simulink model "heli0519"  (R2022a)
settings: Solver=VariableStepAuto  StartTime=0.0  StopTime=5.0  RelTol=1e-3
settings Model: Creator=jixiang  LastModifiedBy=kcx06
settings SolverCC: AlgebraicLoopSolver=TrustRegion
settings DebuggingCC: UnconnectedInputMsg=warning  UnconnectedOutputMsg=warning  UnconnectedLineMsg=warning  SFMachineParentedDataDiag=warning
settings RTWCC: DLArmComputeVersion=19.05

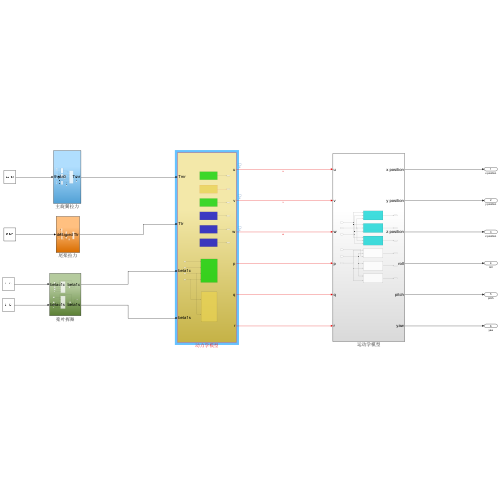
[thumbnail: Simulink's stored preview of the top-level diagram]
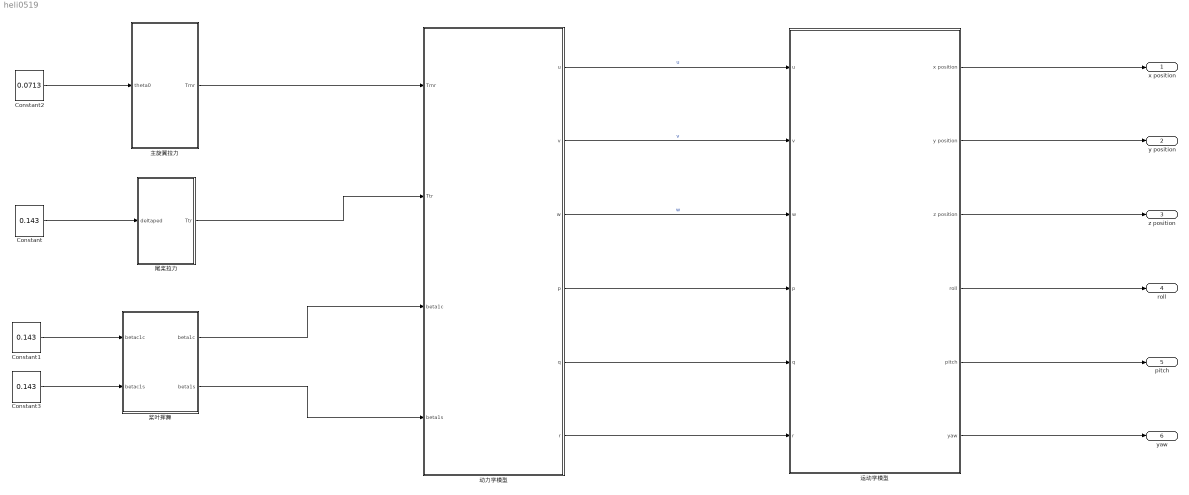
== system heli0519 ==
  Constant : Constant  Value=0.143
  Constant1 : Constant  Value=0.143
  Constant2 : Constant  Value=0.0713
  Constant3 : Constant  Value=0.143
  主旋翼拉力 : Subsystem
  动力学模型 : Subsystem
  尾桨拉力 : Subsystem
  桨叶挥舞 : Subsystem
  运动学模型 : Subsystem
  x position : Outport
  y position : Outport  Port=2
  z position : Outport  Port=3
  roll : Outport  Port=4
  pitch : Outport  Port=5
  yaw : Outport  Port=6
  wires:
  Constant1/1 -> 桨叶挥舞/1(betac1c)
  Constant/1 -> 尾桨拉力/1(deltaped)
  运动学模型/4(roll) -> roll/1
  运动学模型/1(x position) -> x position/1
  动力学模型/1(u) -> 运动学模型/1(u)  "u"
  动力学模型/2(v) -> 运动学模型/2(v)  "v"
  运动学模型/5(pitch) -> pitch/1
  Constant3/1 -> 桨叶挥舞/2(betac1s)
  运动学模型/6(yaw) -> yaw/1
  运动学模型/2(y position) -> y position/1
  动力学模型/4(p) -> 运动学模型/4(p)
  动力学模型/5(q) -> 运动学模型/5(q)
  桨叶挥舞/2(beta1s) -> 动力学模型/4(beta1s)
  动力学模型/6(r) -> 运动学模型/6(r)
  桨叶挥舞/1(beta1c) -> 动力学模型/3(beta1c)
  动力学模型/3(w) -> 运动学模型/3(w)  "w"
  Constant2/1 -> 主旋翼拉力/1(theta0)
  尾桨拉力/1(Ttr) -> 动力学模型/2("Ttr ")
  运动学模型/3(z position) -> z position/1
  主旋翼拉力/1(Tmr) -> 动力学模型/1(Tmr)

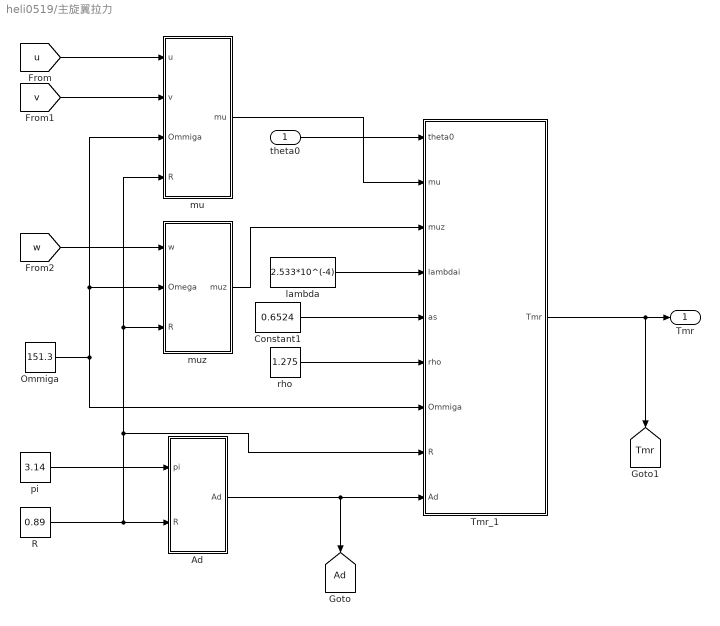
== system heli0519/主旋翼拉力 ==
  theta0 : Inport
  Ad : MATLAB Function  TreatAsAtomicUnit=on
  Constant1 : Constant  Value=0.6524
  Ommiga : Constant  Value=151.3
  R : Constant  Value=0.89
  Tmr_1 : MATLAB Function  TreatAsAtomicUnit=on
  lambda : Constant  Value=2.533*10^(-4)
  mu : MATLAB Function  TreatAsAtomicUnit=on
  muz : MATLAB Function  TreatAsAtomicUnit=on
  pi : Constant  Value=3.14
  rho : Constant  Value=1.275
  Tmr : Outport
  tag scope: Ad=global, Tmr=global
  wires:
  rho/1 -> Tmr_1/6(rho)
  Ommiga/1 -> mu/3(Ommiga), muz/2(Omega), Tmr_1/7(Ommiga)
  mu/1(mu) -> Tmr_1/2(mu)
  R/1 -> mu/4(R), muz/3(R), Tmr_1/8(R), Ad/2(R)
  theta0/1 -> Tmr_1/1(theta0)
  lambda/1 -> Tmr_1/4(lambdai)
  Ad/1(Ad) -> Tmr_1/9(Ad), [Ad]
  Constant1/1 -> Tmr_1/5(as)
  muz/1(muz) -> Tmr_1/3(muz)
  [u] -> mu/1(u)
  [w] -> muz/1(w)
  [v] -> mu/2(v)
  pi/1 -> Ad/1(pi)
  Tmr_1/1(Tmr) -> Tmr/1, [Tmr]

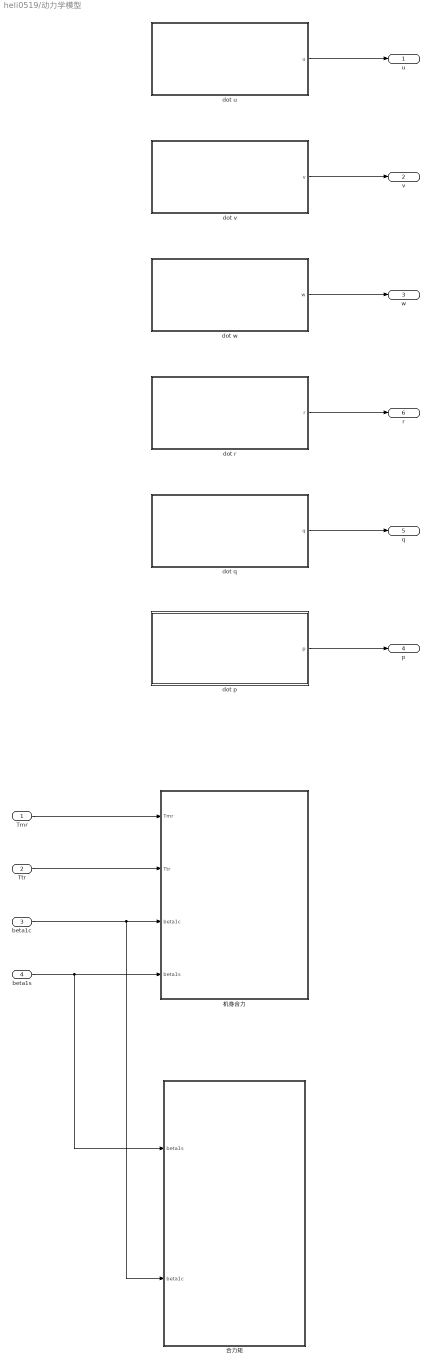
== system heli0519/动力学模型 ==
  Tmr : Inport
  "Ttr " : Inport  Port=2
  beta1c : Inport  Port=3
  beta1s : Inport  Port=4
  dot p : Subsystem
  dot q : Subsystem
  dot r : Subsystem
  dot u : Subsystem
  dot v : Subsystem
  dot w : Subsystem
  合力矩 : Subsystem
  机身合力 : Subsystem
  u : Outport
  v : Outport  Port=2
  w : Outport  Port=3
  p : Outport  Port=4
  q : Outport  Port=5
  r : Outport  Port=6
  wires:
  dot u/1(u) -> u/1
  dot v/1(v) -> v/1
  dot q/1(q) -> q/1
  dot w/1(w) -> w/1
  dot p/1(p) -> p/1
  dot r/1(r) -> r/1
  beta1s/1 -> 合力矩/1(beta1s), 机身合力/4(beta1s)
  "Ttr "/1 -> 机身合力/2(Ttr)
  Tmr/1 -> 机身合力/1(Tmr)
  beta1c/1 -> 合力矩/2(beta1c), 机身合力/3(beta1c)

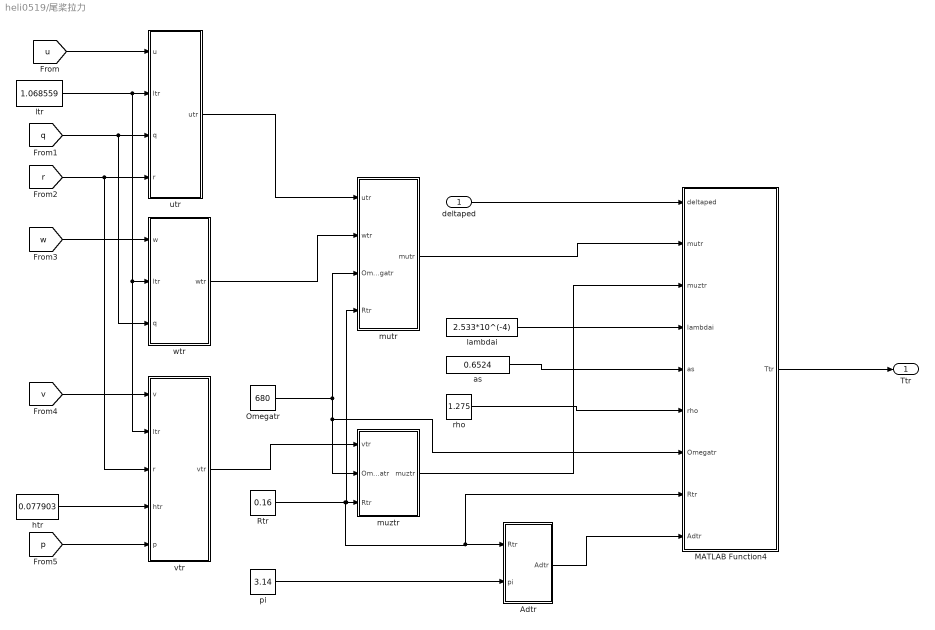
== system heli0519/尾桨拉力 ==
  deltaped : Inport
  Adtr : MATLAB Function  TreatAsAtomicUnit=on
  MATLAB Function4 : MATLAB Function  TreatAsAtomicUnit=on
  Omegatr : Constant  Value=680
  Rtr : Constant  Value=0.16
  as : Constant  Value=0.6524
  htr : Constant  Value=0.077903
  lambdai : Constant  Value=2.533*10^(-4)
  ltr : Constant  Value=1.068559
  mutr : MATLAB Function  TreatAsAtomicUnit=on
  muztr : MATLAB Function  TreatAsAtomicUnit=on
  pi : Constant  Value=3.14
  rho : Constant  Value=1.275
  utr : MATLAB Function  TreatAsAtomicUnit=on
  vtr : MATLAB Function  TreatAsAtomicUnit=on
  wtr : MATLAB Function  TreatAsAtomicUnit=on
  Ttr : Outport
  wires:
  Rtr/1 -> Adtr/1(Rtr), MATLAB Function4/8(Rtr), mutr/4(Rtr), muztr/3(Rtr)
  htr/1 -> vtr/4(htr)
  [p] -> vtr/5(p)
  [q] -> wtr/3(q), utr/3(q)
  deltaped/1 -> MATLAB Function4/1(deltaped)
  Omegatr/1 -> mutr/3(Omegatr), MATLAB Function4/7(Omegatr), muztr/2(Omegatr)
  mutr/1(mutr) -> MATLAB Function4/2(mutr)
  [r] -> vtr/3(r), utr/4(r)
  [u] -> utr/1(u)
  ltr/1 -> vtr/2(ltr), wtr/2(ltr), utr/2(ltr)
  utr/1(utr) -> mutr/1(utr)
  vtr/1(vtr) -> muztr/1(vtr)
  wtr/1(wtr) -> mutr/2(wtr)
  [w] -> wtr/1(w)
  muztr/1(muztr) -> MATLAB Function4/3(muztr)
  lambdai/1 -> MATLAB Function4/4(lambdai)
  as/1 -> MATLAB Function4/5(as)
  rho/1 -> MATLAB Function4/6(rho)
  Adtr/1(Adtr) -> MATLAB Function4/9(Adtr)
  pi/1 -> Adtr/2(pi)
  MATLAB Function4/1(Ttr) -> Ttr/1
  [v] -> vtr/1(v)

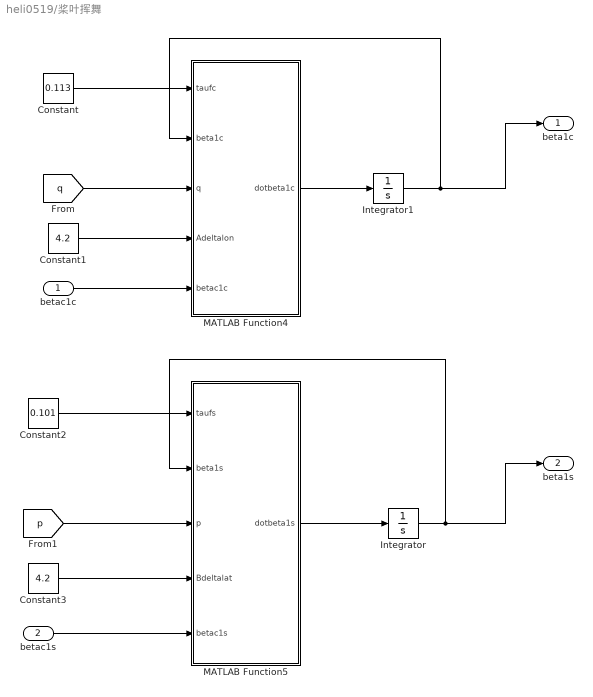
== system heli0519/桨叶挥舞 ==
  betac1c : Inport
  betac1s : Inport  Port=2
  Constant : Constant  Value=0.113
  Constant1 : Constant  Value=4.2
  Constant2 : Constant  Value=0.101
  Constant3 : Constant  Value=4.2
  Integrator : Integrator
  Integrator1 : Integrator
  MATLAB Function4 : MATLAB Function  TreatAsAtomicUnit=on
  MATLAB Function5 : MATLAB Function  TreatAsAtomicUnit=on
  beta1c : Outport
  beta1s : Outport  Port=2
  wires:
  Constant/1 -> MATLAB Function4/1(taufc)
  Integrator/1 -> beta1s/1, MATLAB Function5/2(beta1s)
  betac1c/1 -> MATLAB Function4/5(betac1c)
  [p] -> MATLAB Function5/3(p)
  Constant1/1 -> MATLAB Function4/4(Adeltalon)
  MATLAB Function5/1(dotbeta1s) -> Integrator/1
  Constant2/1 -> MATLAB Function5/1(taufs)
  betac1s/1 -> MATLAB Function5/5(betac1s)
  [q] -> MATLAB Function4/3(q)
  Integrator1/1 -> beta1c/1, MATLAB Function4/2(beta1c)
  MATLAB Function4/1(dotbeta1c) -> Integrator1/1
  Constant3/1 -> MATLAB Function5/4(Bdeltalat)

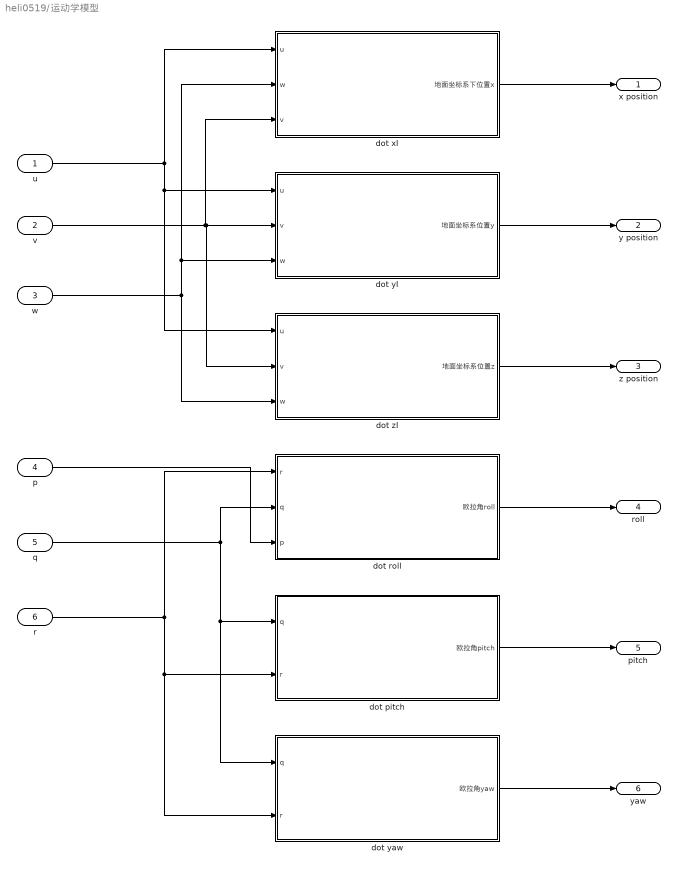
== system heli0519/运动学模型 ==
  u : Inport
  v : Inport  Port=2
  w : Inport  Port=3
  p : Inport  Port=4
  q : Inport  Port=5
  r : Inport  Port=6
  dot pitch : Subsystem
  dot roll : Subsystem
  dot xI : Subsystem
  dot yI : Subsystem
  dot yaw : Subsystem
  dot zI : Subsystem
  x position : Outport
  y position : Outport  Port=2
  z position : Outport  Port=3
  roll : Outport  Port=4
  pitch : Outport  Port=5
  yaw : Outport  Port=6
  wires:
  dot yaw/1(欧拉角yaw) -> yaw/1
  dot yI/1(地面坐标系位置y) -> y position/1
  dot xI/1(地面坐标系下位置x) -> x position/1
  dot roll/1(欧拉角roll) -> roll/1
  dot zI/1(地面坐标系位置z) -> z position/1
  dot pitch/1(欧拉角pitch) -> pitch/1
  u/1 -> dot zI/1(u), dot yI/1(u), dot xI/1(u)
  v/1 -> dot zI/2(v), dot yI/2(v), dot xI/3(v)
  w/1 -> dot zI/3(w), dot yI/3(w), dot xI/2(w)
  r/1 -> dot yaw/2(r), dot pitch/2(r), dot roll/1(r)
  q/1 -> dot yaw/1(q), dot pitch/1(q), dot roll/2(q)
  p/1 -> dot roll/3(p)

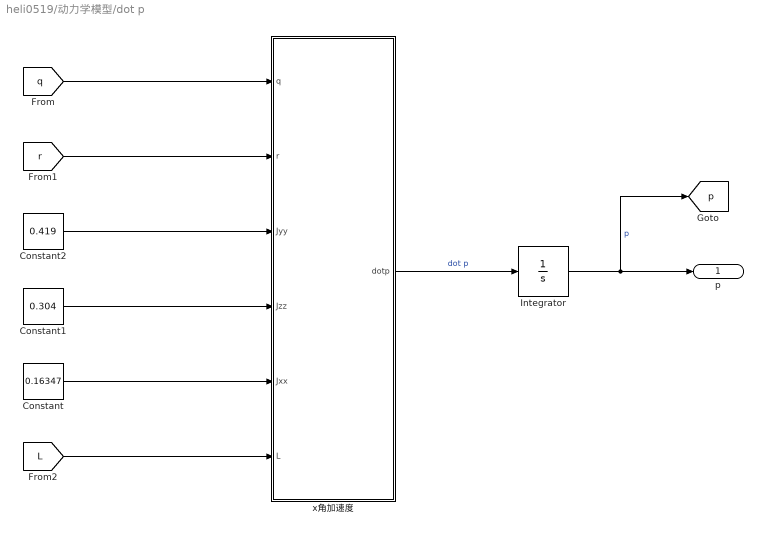
== system heli0519/动力学模型/dot p ==
  Constant : Constant  Value=0.16347
  Constant1 : Constant  Value=0.304
  Constant2 : Constant  Value=0.419
  Integrator : Integrator
  x角加速度 : MATLAB Function  TreatAsAtomicUnit=on
  p : Outport
  tag scope: p=global
  wires:
  x角加速度/1(dotp) -> Integrator/1  "dot p"
  Integrator/1 -> [p], p/1  "p"
  Constant/1 -> x角加速度/5(Jxx)
  Constant2/1 -> x角加速度/3(Jyy)
  Constant1/1 -> x角加速度/4(Jzz)
  [q] -> x角加速度/1(q)
  [r] -> x角加速度/2(r)
  [L] -> x角加速度/6(L)

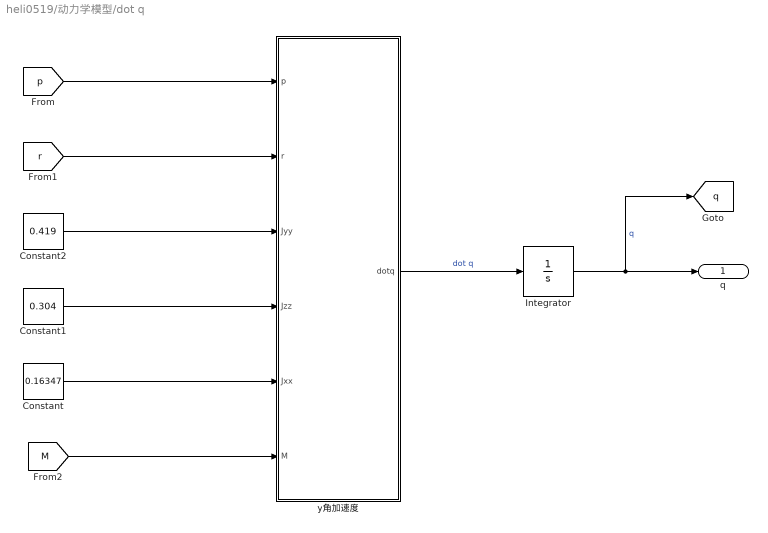
== system heli0519/动力学模型/dot q ==
  Constant : Constant  Value=0.16347
  Constant1 : Constant  Value=0.304
  Constant2 : Constant  Value=0.419
  Integrator : Integrator
  y角加速度 : MATLAB Function  TreatAsAtomicUnit=on
  q : Outport
  tag scope: q=global
  wires:
  Constant1/1 -> y角加速度/4(Jzz)
  Constant2/1 -> y角加速度/3(Jyy)
  Constant/1 -> y角加速度/5(Jxx)
  Integrator/1 -> q/1, [q]  "q"
  y角加速度/1(dotq) -> Integrator/1  "dot q"
  [p] -> y角加速度/1(p)
  [r] -> y角加速度/2(r)
  [M] -> y角加速度/6(M)

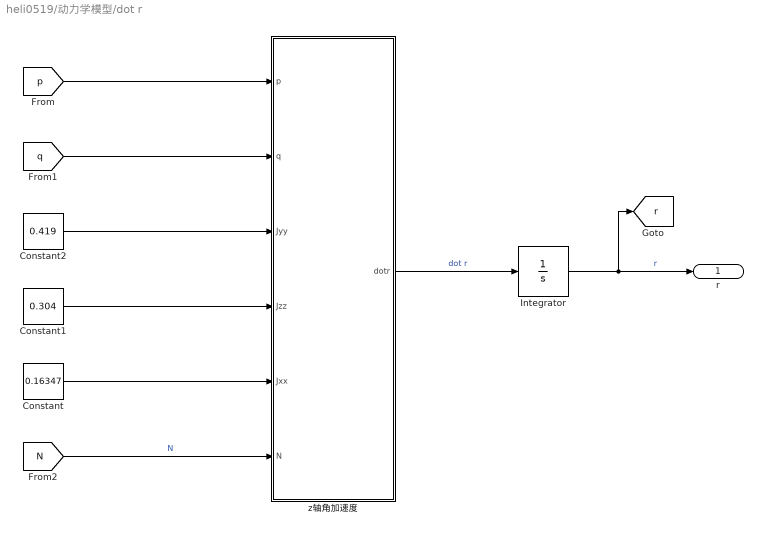
== system heli0519/动力学模型/dot r ==
  Constant : Constant  Value=0.16347
  Constant1 : Constant  Value=0.304
  Constant2 : Constant  Value=0.419
  Integrator : Integrator
  z轴角加速度 : MATLAB Function  TreatAsAtomicUnit=on
  r : Outport
  tag scope: r=global
  wires:
  z轴角加速度/1(dotr) -> Integrator/1  "dot r"
  Integrator/1 -> [r], r/1  "r"
  Constant/1 -> z轴角加速度/5(Jxx)
  Constant2/1 -> z轴角加速度/3(Jyy)
  Constant1/1 -> z轴角加速度/4(Jzz)
  [p] -> z轴角加速度/1(p)
  [q] -> z轴角加速度/2(q)
  [N] -> z轴角加速度/6(N)  "N"

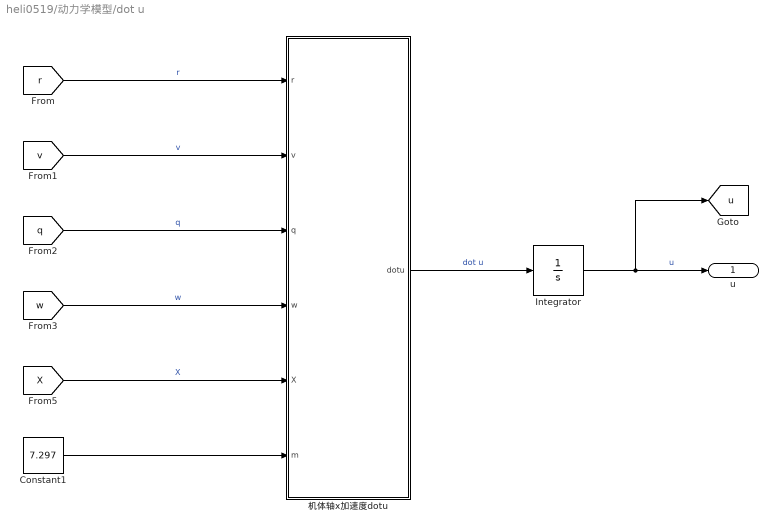
== system heli0519/动力学模型/dot u ==
  Constant1 : Constant  Value=7.297
  Integrator : Integrator
  机体轴x加速度dotu : MATLAB Function  TreatAsAtomicUnit=on
  u : Outport
  tag scope: u=global
  wires:
  Constant1/1 -> 机体轴x加速度dotu/6(m)
  Integrator/1 -> [u], u/1  "u"
  机体轴x加速度dotu/1(dotu) -> Integrator/1  "dot u"
  [r] -> 机体轴x加速度dotu/1(r)  "r"
  [v] -> 机体轴x加速度dotu/2(v)  "v"
  [q] -> 机体轴x加速度dotu/3(q)  "q"
  [w] -> 机体轴x加速度dotu/4(w)  "w"
  [X] -> 机体轴x加速度dotu/5(X)  "X"

== system heli0519/动力学模型/dot v ==
  Constant1 : Constant  Value=7.297
  Integrator : Integrator
  机体轴y加速度dotv : MATLAB Function  TreatAsAtomicUnit=on
  v : Outport
  tag scope: v=global
  wires:
  机体轴y加速度dotv/1(dotv) -> Integrator/1  "dot v"
  Integrator/1 -> [v], v/1  "v"
  Constant1/1 -> 机体轴y加速度dotv/6(m)
  [p] -> 机体轴y加速度dotv/1(p)
  [w] -> 机体轴y加速度dotv/2(w)
  [r] -> 机体轴y加速度dotv/3(r)
  [u] -> 机体轴y加速度dotv/4(u)
  [Y] -> 机体轴y加速度dotv/5(Y)

== system heli0519/动力学模型/dot w ==
  Constant1 : Constant  Value=7.297
  Integrator : Integrator
  机体轴z加速度dotw : MATLAB Function  TreatAsAtomicUnit=on
  w : Outport
  tag scope: w=global
  wires:
  Constant1/1 -> 机体轴z加速度dotw/6(m)
  Integrator/1 -> [w], w/1  "w"
  机体轴z加速度dotw/1(dotw) -> Integrator/1  "dot w"
  [q] -> 机体轴z加速度dotw/1(q)
  [u] -> 机体轴z加速度dotw/2(u)
  [p] -> 机体轴z加速度dotw/3(p)
  [v] -> 机体轴z加速度dotw/4(v)
  [Z] -> 机体轴z加速度dotw/5(Z)

== system heli0519/动力学模型/合力矩 ==
  beta1s : Inport
  beta1c : Inport  Port=2
  MATLAB Function : MATLAB Function  TreatAsAtomicUnit=on
  MATLAB Function1 : MATLAB Function  TreatAsAtomicUnit=on
  主旋翼力矩 : Subsystem
  尾桨力矩 : Subsystem
  tag scope: L=global, M=global, N=global
  wires:
  beta1s/1 -> 主旋翼力矩/1(beta1s)
  beta1c/1 -> 主旋翼力矩/2(beta1c)
  MATLAB Function1/1(N) -> [N]
  MATLAB Function/1(L) -> [L]
  主旋翼力矩/2(Mmr) -> [M]
  主旋翼力矩/1(Lmr) -> MATLAB Function/1(Lmr)
  尾桨力矩/1(Ltr) -> MATLAB Function/2(Ltr)
  主旋翼力矩/3(Nmr) -> MATLAB Function1/1(Nmr)
  尾桨力矩/2(Ntr) -> MATLAB Function1/2(Ntr)

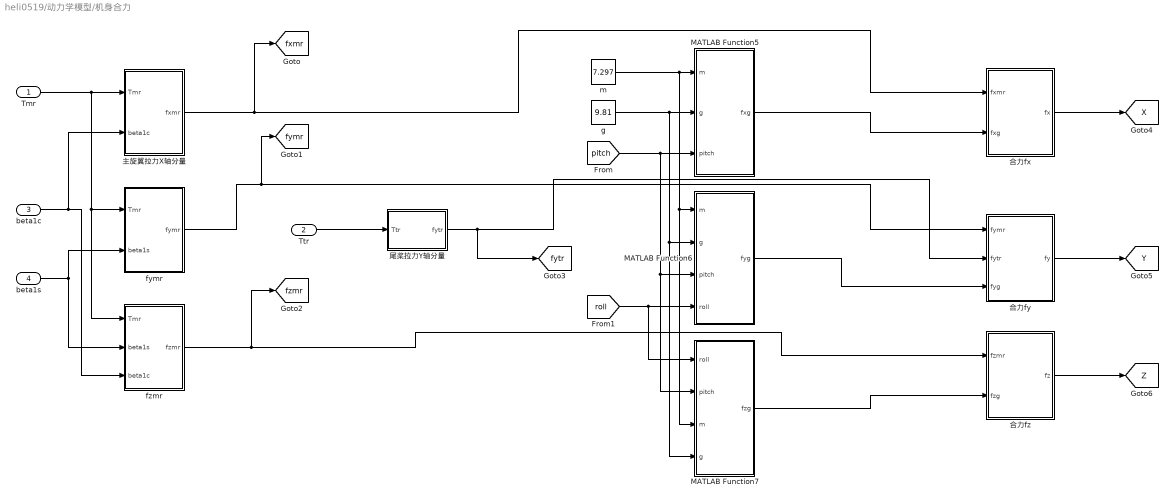
== system heli0519/动力学模型/机身合力 ==
  Tmr : Inport
  Ttr : Inport  Port=2
  beta1c : Inport  Port=3
  beta1s : Inport  Port=4
  MATLAB Function5 : MATLAB Function  TreatAsAtomicUnit=on
  MATLAB Function6 : MATLAB Function  TreatAsAtomicUnit=on
  MATLAB Function7 : MATLAB Function  TreatAsAtomicUnit=on
  fymr : MATLAB Function  TreatAsAtomicUnit=on
  fzmr : MATLAB Function  TreatAsAtomicUnit=on
  g : Constant  Value=9.81
  m : Constant  Value=7.297
  主旋翼拉力X轴分量 : MATLAB Function  TreatAsAtomicUnit=on
  合力fx : MATLAB Function  TreatAsAtomicUnit=on
  合力fy : MATLAB Function  TreatAsAtomicUnit=on
  合力fz : MATLAB Function  TreatAsAtomicUnit=on
  尾桨拉力Y轴分量 : MATLAB Function  TreatAsAtomicUnit=on
  tag scope: X=global, Y=global, Z=global, fxmr=global, fymr=global, fytr=global, fzmr=global
  wires:
  MATLAB Function7/1(fzg) -> 合力fz/2(fzg)
  Tmr/1 -> 主旋翼拉力X轴分量/1(Tmr), fzmr/1(Tmr), fymr/1(Tmr)
  MATLAB Function5/1(fxg) -> 合力fx/2(fxg)
  g/1 -> MATLAB Function7/4(g), MATLAB Function6/2(g), MATLAB Function5/2(g)
  fymr/1(fymr) -> [fymr], 合力fy/1(fymr)
  [pitch] -> MATLAB Function7/2(pitch), MATLAB Function6/3(pitch), MATLAB Function5/3(pitch)
  [roll] -> MATLAB Function7/1(roll), MATLAB Function6/4(roll)
  fzmr/1(fzmr) -> [fzmr], 合力fz/1(fzmr)
  beta1s/1 -> fzmr/2(beta1s), fymr/2(beta1s)
  尾桨拉力Y轴分量/1(fytr) -> [fytr], 合力fy/2(fytr)
  beta1c/1 -> fzmr/3(beta1c), 主旋翼拉力X轴分量/2(beta1c)
  m/1 -> MATLAB Function7/3(m), MATLAB Function6/1(m), MATLAB Function5/1(m)
  Ttr/1 -> 尾桨拉力Y轴分量/1(Ttr)
  主旋翼拉力X轴分量/1(fxmr) -> [fxmr], 合力fx/1(fxmr)
  MATLAB Function6/1(fyg) -> 合力fy/3(fyg)
  合力fx/1(fx) -> [X]
  合力fz/1(fz) -> [Z]
  合力fy/1(fy) -> [Y]

== system heli0519/运动学模型/dot pitch ==
  q : Inport
  r : Inport  Port=2
  Integrator : Integrator
  pitch欧拉角速度 : MATLAB Function  TreatAsAtomicUnit=on
  欧拉角pitch : Outport
  tag scope: pitch=global
  wires:
  Integrator/1 -> [pitch], 欧拉角pitch/1
  pitch欧拉角速度/1(dotpitch) -> Integrator/1  "dot pitchl"
  q/1 -> pitch欧拉角速度/1(q)
  r/1 -> pitch欧拉角速度/2(r)
  [roll] -> pitch欧拉角速度/3(roll)

== system heli0519/运动学模型/dot roll ==
  r : Inport
  q : Inport  Port=2
  p : Inport  Port=3
  Integrator : Integrator
  roll欧拉角速度 : MATLAB Function  TreatAsAtomicUnit=on
  欧拉角roll : Outport
  tag scope: roll=global
  wires:
  roll欧拉角速度/1(dotroll) -> Integrator/1  "dot roll"
  Integrator/1 -> roll欧拉角速度/4(roll), [roll], 欧拉角roll/1  "roll"
  p/1 -> roll欧拉角速度/1(p)
  q/1 -> roll欧拉角速度/2(q)
  r/1 -> roll欧拉角速度/3(r)
  [pitch] -> roll欧拉角速度/5(pitch)

== system heli0519/运动学模型/dot xI ==
  u : Inport
  w : Inport  Port=2
  v : Inport  Port=3
  Integrator : Integrator
  地面坐标系下x速度 : MATLAB Function  TreatAsAtomicUnit=on
  地面坐标系下位置x : Outport
  wires:
  u/1 -> 地面坐标系下x速度/4(u)
  [yaw] -> 地面坐标系下x速度/3(yaw)
  v/1 -> 地面坐标系下x速度/5(v)
  Integrator/1 -> 地面坐标系下位置x/1  "x position"
  地面坐标系下x速度/1(dotx) -> Integrator/1  "dot x"
  [pitch] -> 地面坐标系下x速度/1(pitch)
  [roll] -> 地面坐标系下x速度/2(roll)
  w/1 -> 地面坐标系下x速度/6(w)

== system heli0519/运动学模型/dot yI ==
  u : Inport
  v : Inport  Port=2
  w : Inport  Port=3
  Integrator : Integrator
  地面坐标系y速度 : MATLAB Function  TreatAsAtomicUnit=on
  地面坐标系位置y : Outport
  wires:
  地面坐标系y速度/1(doty) -> Integrator/1  "dot y"
  Integrator/1 -> 地面坐标系位置y/1  "y position"
  [pitch] -> 地面坐标系y速度/1(pitch)
  [roll] -> 地面坐标系y速度/2(roll)
  [yaw] -> 地面坐标系y速度/3(yaw)
  u/1 -> 地面坐标系y速度/4(u)
  v/1 -> 地面坐标系y速度/5(v)
  w/1 -> 地面坐标系y速度/6(w)

== system heli0519/运动学模型/dot yaw ==
  q : Inport
  r : Inport  Port=2
  Integrator : Integrator
  yaw欧拉角速度 : MATLAB Function  TreatAsAtomicUnit=on
  欧拉角yaw : Outport
  tag scope: yaw=global
  wires:
  yaw欧拉角速度/1(dotyaw) -> Integrator/1  "dot yaw"
  Integrator/1 -> [yaw], 欧拉角yaw/1
  q/1 -> yaw欧拉角速度/1(q)
  r/1 -> yaw欧拉角速度/2(r)
  [roll] -> yaw欧拉角速度/3(roll)
  [pitch] -> yaw欧拉角速度/4(pitch)

== system heli0519/运动学模型/dot zI ==
  u : Inport
  v : Inport  Port=2
  w : Inport  Port=3
  Integrator : Integrator
  地面坐标系加速度z : MATLAB Function  TreatAsAtomicUnit=on
  地面坐标系位置z : Outport
  wires:
  Integrator/1 -> 地面坐标系位置z/1  "z position"
  地面坐标系加速度z/1(dotz) -> Integrator/1  "dot zI"
  [pitch] -> 地面坐标系加速度z/1(pitch)
  [roll] -> 地面坐标系加速度z/2(roll)
  u/1 -> 地面坐标系加速度z/3(u)
  v/1 -> 地面坐标系加速度z/4(v)
  w/1 -> 地面坐标系加速度z/5(w)

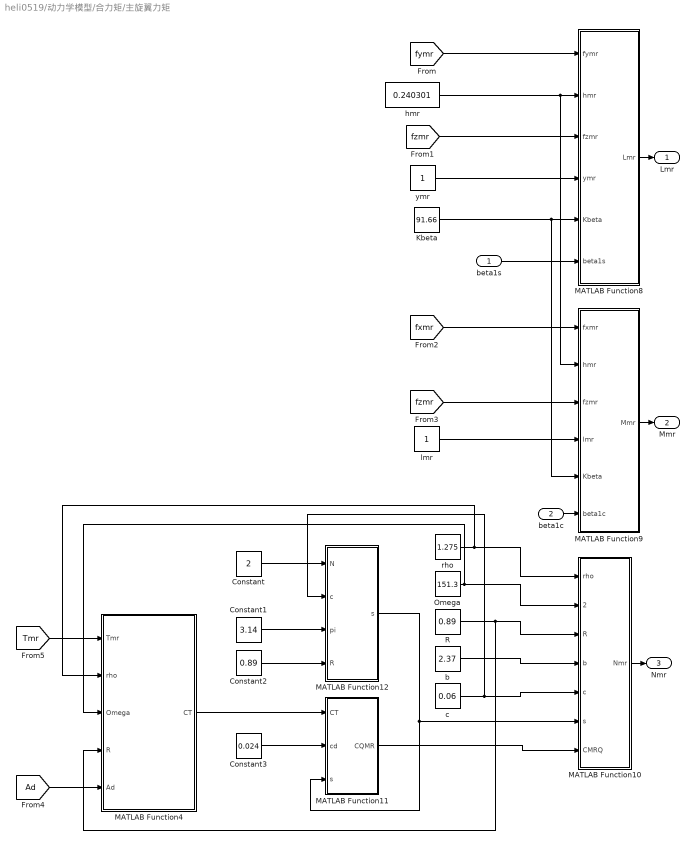
== system heli0519/动力学模型/合力矩/主旋翼力矩 ==
  beta1s : Inport
  beta1c : Inport  Port=2
  Constant : Constant  Value=2
  Constant1 : Constant  Value=3.14
  Constant2 : Constant  Value=0.89
  Constant3 : Constant  Value=0.024
  Kbeta : Constant  Value=91.66
  MATLAB Function10 : MATLAB Function  TreatAsAtomicUnit=on
  MATLAB Function11 : MATLAB Function  TreatAsAtomicUnit=on
  MATLAB Function12 : MATLAB Function  TreatAsAtomicUnit=on
  MATLAB Function4 : MATLAB Function  TreatAsAtomicUnit=on
  MATLAB Function8 : MATLAB Function  TreatAsAtomicUnit=on
  MATLAB Function9 : MATLAB Function  TreatAsAtomicUnit=on
  Omega : Constant  Value=151.3
  R : Constant  Value=0.89
  b : Constant  Value=2.37
  c : Constant  Value=0.06
  hmr : Constant  Value=0.240301
  lmr : Constant
  rho : Constant  Value=1.275
  ymr : Constant
  Lmr : Outport
  Mmr : Outport  Port=2
  Nmr : Outport  Port=3
  wires:
  R/1 -> MATLAB Function4/4(R), MATLAB Function10/3(R)
  rho/1 -> MATLAB Function4/2(rho), MATLAB Function10/1(rho)
  Constant2/1 -> MATLAB Function12/4(R)
  Constant1/1 -> MATLAB Function12/3(pi)
  [fxmr] -> MATLAB Function9/1(fxmr)
  Constant3/1 -> MATLAB Function11/2(cd)
  [Tmr] -> MATLAB Function4/1(Tmr)
  Constant/1 -> MATLAB Function12/1(N)
  MATLAB Function11/1(CQMR) -> MATLAB Function10/7(CMRQ)
  MATLAB Function12/1(s) -> MATLAB Function10/6(s), MATLAB Function11/3(s)
  Kbeta/1 -> MATLAB Function9/5(Kbeta), MATLAB Function8/5(Kbeta)
  [fzmr] -> MATLAB Function8/3(fzmr)
  [fymr] -> MATLAB Function8/1(fymr)
  hmr/1 -> MATLAB Function9/2(hmr), MATLAB Function8/2(hmr)
  ymr/1 -> MATLAB Function8/4(ymr)
  [Ad] -> MATLAB Function4/5(Ad)
  [fzmr] -> MATLAB Function9/3(fzmr)
  lmr/1 -> MATLAB Function9/4(lmr)
  b/1 -> MATLAB Function10/4(b)
  MATLAB Function9/1(Mmr) -> Mmr/1
  MATLAB Function10/1(Nmr) -> Nmr/1
  c/1 -> MATLAB Function12/2(c), MATLAB Function10/5(c)
  Omega/1 -> MATLAB Function4/3(Omega), MATLAB Function10/2(Omega)
  MATLAB Function4/1(CT) -> MATLAB Function11/1(CT)
  MATLAB Function8/1(Lmr) -> Lmr/1
  beta1c/1 -> MATLAB Function9/6(beta1c)
  beta1s/1 -> MATLAB Function8/6(beta1s)

== system heli0519/动力学模型/合力矩/尾桨力矩 ==
  MATLAB Function4 : MATLAB Function  TreatAsAtomicUnit=on
  MATLAB Function5 : MATLAB Function  TreatAsAtomicUnit=on
  htr : Constant  Value=0.077903
  ltr : Constant  Value=1.068599
  Ltr : Outport
  Ntr : Outport  Port=2
  wires:
  [fytr] -> MATLAB Function5/1(fytr), MATLAB Function4/1(fytr)
  MATLAB Function5/1(Ntr) -> Ntr/1
  htr/1 -> MATLAB Function4/2(htr)
  ltr/1 -> MATLAB Function5/2(ltr)
  MATLAB Function4/1(Ltr) -> Ltr/1

== matlab function heli0519/运动学模型/dot yI/地面坐标系y速度 ==
  data: pitch input; roll input; yaw input; u input; doty output; v input; w input
function doty = fcn(pitch,roll,yaw,u,v,w)

doty = cos(pitch)*cos(yaw)*u+(cos(roll)*cos(yaw)+sin(roll)*sin(yaw)*sin(pitch))*v+(cos(pitch)*sin(yaw)*sin(roll)-cos(yaw)*sin(roll))*w;

== matlab function heli0519/运动学模型/dot zI/地面坐标系加速度z ==
  data: pitch input; roll input; u input; dotz output; v input; w input
function dotz = fcn(pitch,roll,u,v,w)

dotz =-sin(pitch)*u+cos(pitch)*sin(roll)*v+cos(roll)*cos(pitch)*w;

== matlab function heli0519/运动学模型/dot roll/roll欧拉角速度 ==
  data: p input; q input; r input; roll input; pitch input; dotroll output
function dotroll = fcn(p,q,r,roll,pitch)

dotroll = p+sin(roll)*tan(pitch)*q+cos(roll)*tan(pitch)*r;

== matlab function heli0519/运动学模型/dot pitch/pitch欧拉角速度 ==
  data: q input; r input; roll input; dotpitch output
function dotpitch = fcn(q,r,roll)

dotpitch = cos(roll)*q-sin(roll)*r;

== matlab function heli0519/运动学模型/dot yaw/yaw欧拉角速度 ==
  data: q input; r input; roll input; dotyaw output; pitch input
function dotyaw = fcn(q,r,roll,pitch)

dotyaw = (sin(roll)/cos(pitch))*q+(cos(roll)/cos(pitch))*r;

== matlab function heli0519/动力学模型/合力矩/MATLAB Function ==
  data: Lmr input; L output; Ltr input
function L = fcn(Lmr,Ltr)

L = Lmr+Ltr;

== matlab function heli0519/动力学模型/dot v/机体轴y加速度dotv ==
  data: p input; w input; r input; dotv output; u input; Y input; m input
function dotv = fcn(p,w,r,u,Y,m)

dotv = p*w-r*u+Y/m;

== matlab function heli0519/动力学模型/合力矩/MATLAB Function1 ==
  data: Nmr input; N output; Ntr input
function N = fcn(Nmr,Ntr)

N = Nmr+Ntr;

== matlab function heli0519/桨叶挥舞/MATLAB Function4 ==
  data: taufc input; dotbeta1c output; beta1c input; q input; Adeltalon input; betac1c input
function dotbeta1c = fcn(taufc,beta1c,q,Adeltalon,betac1c)

dotbeta1c = -beta1c/taufc-q+Adeltalon*betac1c/taufc

== matlab function heli0519/桨叶挥舞/MATLAB Function5 ==
  data: taufs input; dotbeta1s output; beta1s input; p input; Bdeltalat input; betac1s input
function dotbeta1s = fcn(taufs,beta1s,p,Bdeltalat,betac1s)

dotbeta1s = -beta1s/taufs-p+Bdeltalat*betac1s/taufs;

== matlab function heli0519/主旋翼拉力/Tmr_1 ==
  data: theta0 input; Tmr output; mu input; muz input; lambdai input; as input; rho input; Ommiga input; R input; Ad input
function Tmr = fcn(theta0,mu,muz,lambdai,as,rho,Ommiga,R,Ad)

Tmr = (theta0*(1/3+mu^2/2)-(muz+lambdai)/2)*(as/2)*rho*Ommiga^2*R^2*Ad;

== matlab function heli0519/主旋翼拉力/mu ==
  data: u input; mu output; v input; Ommiga input; R input
function mu = fcn(u,v,Ommiga,R)

mu = ((u^2+v^2)^0.5)/(Ommiga*R);

== matlab function heli0519/主旋翼拉力/muz ==
  data: w input; muz output; Omega input; R input
function muz = fcn(w,Omega,R)

muz = w/(Omega*R);

== matlab function heli0519/主旋翼拉力/Ad ==
  data: pi input; Ad output; R input
function Ad = fcn(pi,R)

Ad = pi*R^2;

== matlab function heli0519/尾桨拉力/MATLAB Function4 ==
  data: deltaped input; Ttr output; mutr input; muztr input; lambdai input; as input; rho input; Omegatr input; Rtr input; Adtr input
function Ttr = fcn(deltaped,mutr,muztr,lambdai,as,rho,Omegatr,Rtr,Adtr)

Ttr = (deltaped*(1/3+mutr^2/2)-(muztr+lambdai))*as*rho*Omegatr^2*Rtr^2*Adtr/2;

== matlab function heli0519/尾桨拉力/muztr ==
  data: vtr input; muztr output; Omegatr input; Rtr input
function muztr = fcn(vtr,Omegatr,Rtr)

muztr = vtr/Omegatr*Rtr;

== matlab function heli0519/尾桨拉力/vtr ==
  data: v input; vtr output; ltr input; r input; htr input; p input
function vtr = fcn(v,ltr,r,htr,p)

vtr = v-ltr*r-htr*abs(p);

== matlab function heli0519/尾桨拉力/wtr ==
  data: w input; wtr output; ltr input; q input
function wtr = fcn(w,ltr,q)

wtr = w-ltr*q;

== matlab function heli0519/尾桨拉力/utr ==
  data: u input; utr output; ltr input; q input; r input
function utr = fcn(u,ltr,q,r)

utr = u+abs(ltr*q+ltr*r);

== matlab function heli0519/动力学模型/dot u/机体轴x加速度dotu ==
  data: r input; dotu output; v input; q input; w input; X input; m input
function dotu = fcn(r,v,q,w,X,m)

dotu = r*v-q*w+X/m;

== matlab function heli0519/尾桨拉力/mutr ==
  data: utr input; mutr output; wtr input; Omegatr input; Rtr input
function mutr = fcn(utr,wtr,Omegatr,Rtr)

mutr = (utr^2+wtr^2)^0.5/(Omegatr*Rtr);

== matlab function heli0519/尾桨拉力/Adtr ==
  data: Rtr input; pi input; Adtr output
function Adtr = fcn(Rtr,pi)

Adtr = pi*Rtr^2;

== matlab function heli0519/动力学模型/机身合力/主旋翼拉力X轴分量 ==
  data: Tmr input; fxmr output; beta1c input
function fxmr = fcn(Tmr,beta1c)

fxmr = -Tmr*sin(beta1c)*cos(beta1c);

== matlab function heli0519/动力学模型/机身合力/fymr ==
  data: Tmr input; fymr output; beta1s input
function fymr = fcn(Tmr,beta1s)

fymr = Tmr*sin(beta1s)*cos(beta1s);

== matlab function heli0519/动力学模型/机身合力/fzmr ==
  data: Tmr input; fzmr output; beta1s input; beta1c input
function fzmr = fcn(Tmr,beta1s,beta1c)

fzmr = -Tmr*cos(beta1s)*cos(beta1c);

== matlab function heli0519/动力学模型/机身合力/尾桨拉力Y轴分量 ==
  data: Ttr input; fytr output
function fytr = fcn(Ttr)

fytr = -Ttr;

== matlab function heli0519/动力学模型/机身合力/MATLAB Function5 ==
  data: m input; fxg output; g input; pitch input
function fxg = fcn(m,g,pitch)

fxg = -sin(pitch)*m*g;

== matlab function heli0519/动力学模型/机身合力/MATLAB Function6 ==
  data: m input; fyg output; g input; pitch input; roll input
function fyg = fcn(m,g,pitch,roll)

fyg = sin(roll)*cos(pitch)*m*g;

== matlab function heli0519/动力学模型/机身合力/MATLAB Function7 ==
  data: roll input; fzg output; pitch input; m input; g input
function fzg = fcn(roll,pitch,m,g)

fzg = cos(roll)*cos(pitch)*m*g;

== matlab function heli0519/动力学模型/合力矩/主旋翼力矩/MATLAB Function8 ==
  data: fymr input; Lmr output; hmr input; fzmr input; ymr input; Kbeta input; beta1s input
function Lmr = fcn(fymr,hmr,fzmr,ymr,Kbeta,beta1s)

Lmr = fymr*hmr-fzmr*ymr+Kbeta*beta1s;

== matlab function heli0519/动力学模型/合力矩/主旋翼力矩/MATLAB Function9 ==
  data: fxmr input; Mmr output; hmr input; fzmr input; lmr input; Kbeta input; beta1c input
function Mmr = fcn(fxmr,hmr,fzmr,lmr,Kbeta,beta1c)

Mmr = fxmr*hmr+fzmr*lmr+Kbeta*beta1c;

== matlab function heli0519/动力学模型/合力矩/主旋翼力矩/MATLAB Function10 ==
  data: rho input; Nmr output; Omega input; R input; b input; c input; s input; CMRQ input
function Nmr = fcn(rho,Omega,R,b,c,s,CMRQ)

Nmr = -rho*Omega^2*R^2*b*c*R^2*CMRQ/s;

== matlab function heli0519/动力学模型/dot w/机体轴z加速度dotw ==
  data: q input; u input; p input; v input; dotw output; Z input; m input
function dotw = fcn(q,u,p,v,Z,m)

dotw = q*u-p*v+Z/m;

== matlab function heli0519/动力学模型/合力矩/主旋翼力矩/MATLAB Function11 ==
  data: CT input; CQMR output; cd input; s input
function CQMR = fcn(CT,cd,s)

CQMR = CT*(CT/2)^2+cd*s/8;

== matlab function heli0519/动力学模型/合力矩/主旋翼力矩/MATLAB Function12 ==
  data: N input; s output; c input; pi input; R input
function s = fcn(N,c,pi,R)

s = N*c/(pi*R);

== matlab function heli0519/动力学模型/机身合力/合力fx ==
  data: fxmr input; fx output; fxg input
function fx = fcn(fxmr,fxg)

fx = fxmr+fxg;

== matlab function heli0519/动力学模型/机身合力/合力fy ==
  data: fymr input; fy output; fytr input; fyg input
function fy = fcn(fymr,fytr,fyg)

fy = fymr+fytr+fyg;

== matlab function heli0519/动力学模型/机身合力/合力fz ==
  data: fzmr input; fz output; fzg input
function fz = fcn(fzmr,fzg)

fz = fzmr+fzg;

== matlab function heli0519/动力学模型/合力矩/主旋翼力矩/MATLAB Function4 ==
  data: Tmr input; CT output; rho input; Omega input; R input; Ad input
function CT = fcn(Tmr,rho,Omega,R,Ad)

CT = Tmr/(rho*Omega^2*R^2*Ad);

== matlab function heli0519/动力学模型/合力矩/尾桨力矩/MATLAB Function4 ==
  data: fytr input; Ltr output; htr input
function Ltr = fcn(fytr,htr)

Ltr = fytr*htr;

== matlab function heli0519/动力学模型/合力矩/尾桨力矩/MATLAB Function5 ==
  data: fytr input; Ntr output; ltr input
function Ntr = fcn(fytr,ltr)

Ntr = -fytr*ltr;

== matlab function heli0519/动力学模型/dot p/x角加速度 ==
  data: q input; r input; Jyy input; Jzz input; dotp output; Jxx input; L input
function dotp = fcn(q,r,Jyy,Jzz,Jxx,L)

dotp = q*r*(Jyy-Jzz)/Jxx+L/Jxx;

== matlab function heli0519/动力学模型/dot q/y角加速度 ==
  data: p input; r input; Jyy input; Jzz input; dotq output; Jxx input; M input
function dotq = fcn(p,r,Jyy,Jzz,Jxx,M)

dotq = p*r*(Jzz-Jxx)/Jyy+M/Jyy;

== matlab function heli0519/动力学模型/dot r/z轴角加速度 ==
  data: p input; q input; Jyy input; Jzz input; dotr output; Jxx input; N input
function dotr = fcn(p,q,Jyy,Jzz,Jxx,N)

dotr = q*p*(Jxx-Jyy)/Jzz+N/Jzz;

== matlab function heli0519/运动学模型/dot xI/地面坐标系下x速度 ==
  data: pitch input; roll input; yaw input; u input; dotx output; v input; w input
function dotx = fcn(pitch,roll,yaw,u,v,w)

dotx = cos(pitch)*cos(yaw)*u+(sin(pitch)*sin(roll)*cos(yaw)-cos(roll)*sin(yaw))*v+(sin(pitch)*cos(roll)*cos(yaw)+sin(roll)*sin(yaw))*w;
